simulink model "task1_lab2"  (R2020b)
settings: Solver=ode45  StartTime=1  StopTime=2  MaxStep=0.02  RelTol=1e-3  EnableMultiTasking=on
settings Model: Creator=JackShen  LastModifiedBy=mluser
settings DataIOCC: LimitDataPoints=on  ReturnWorkspaceOutputs=off
settings OptimizationCC: LifeSpan=inf
settings DebuggingCC: AllowSymbolicDim=off  SFUnexpectedBacktrackingDiag=warning  SFNoUnconditionalDefaultTransitionDiag=warning  SFExecutionAtInitializationDiag=none  ArithmeticOperatorsInVariantConditions=warning
settings ModelReferenceCC: PropagateSignalLabelsOutOfModel=off
settings SFSimCC: SimUseLocalCustomCode=off  CustomCodeUndefinedFunction=UseInterfaceOnly
settings RTWCC: RTWUseLocalCustomCode=off
settings CodeAppCC: StateflowObjectComments=on
settings GRTTargetCC: TargetLangStandard=C89/C90 (ANSI)
settings ConfigComp: CovMetricSettings=dw  CovSaveCumulativeToWorkspaceVar=on  CovSaveSingleToWorkspaceVar=on  CovExternalEMLEnable=off

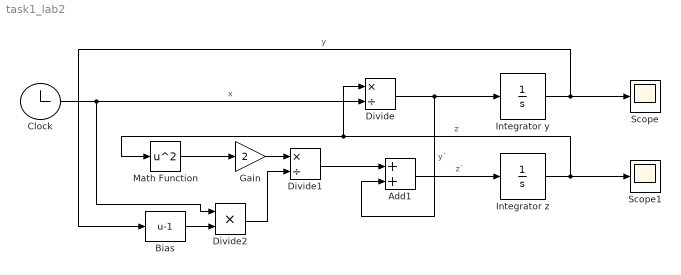
== system task1_lab2 ==
  Add1 : Sum
  Bias : Bias  Bias=-1
  Clock : Clock
  Divide : Product  Inputs=*/
  Divide1 : Product  Inputs=*/
  Divide2 : Product  Inputs=**
  Gain : Gain  Gain=2
  Integrator y : Integrator
  Integrator z : Integrator  InitialCondition=0.33
  Math Function : Math  Operator=square  SignedPower=on  SaturateOnIntegerOverflow=on
  Scope : Scope
  Scope1 : Scope
  wires:
  Divide1/1 -> Add1/1
  Divide/1 -> Add1/2, Integrator y/1  "y`"
  Integrator z/1 -> Math Function/1, Divide/1, Scope1/1  "z"
  Divide2/1 -> Divide1/2
  Add1/1 -> Integrator z/1  "z`"
  Bias/1 -> Divide2/2
  Clock/1 -> Divide/2, Divide2/1  "x"
  Integrator y/1 -> Bias/1, Scope/1  "y"
  Math Function/1 -> Gain/1
  Gain/1 -> Divide1/1
